simulink model "ps1"  (R2020b)
settings: Solver=VariableStepAuto  StartTime=0.0  StopTime=10.0  RelTol=1e-3
undefined symbols (not defined in the file): b, K1, k12, M1, M2
settings Model: Creator=prana  LastModifiedBy=prana

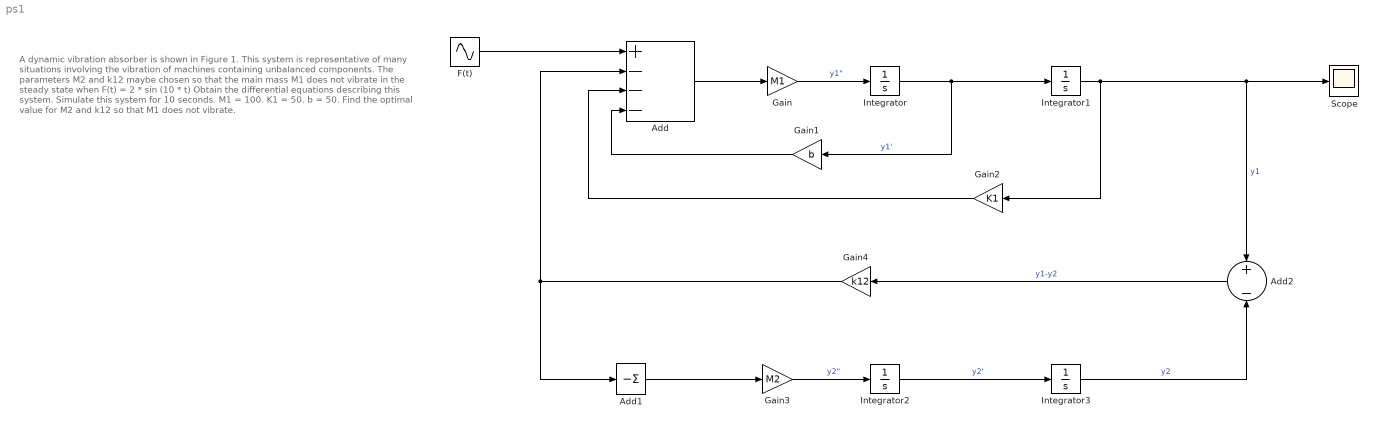
== system ps1 ==
  note: A dynamic vibration absorber is shown in Figure 1. This system is representative of many situations involving the vibration of machines containing unbalanced components. The parameters M2 and k12 maybe chosen so that the main mass M1 does not vibrate in the steady state when F(t) = 2 * sin (10 * t) Obtain the differential equations describing this system. Simulate this system for 10 seconds. M1 = 100. K1 = 50. b = 50. Find the optimal value for M2 and k12 so that M1 does not vibrate.
  Add : Sum  Inputs=+---
  Add1 : Sum  Inputs=-
  Add2 : Sum  Inputs=+-
  F(t) : Sin  Amplitude=2  Frequency=10  SampleTime=0
  Gain : Gain  Gain=M1
  Gain1 : Gain  Gain=b
  Gain2 : Gain  Gain=K1
  Gain3 : Gain  Gain=M2
  Gain4 : Gain  Gain=k12
  Integrator{,1..3} (4 alike) : Integrator
  Scope : Scope
  wires:
  Integrator/1 -> Gain1/1, Integrator1/1  "y1'"
  Gain/1 -> Integrator/1  "y1\""
  Add/1 -> Gain/1
  F(t)/1 -> Add/1
  Integrator1/1 -> Gain2/1, Scope/1, Add2/1  "y1"
  Gain1/1 -> Add/4
  Gain2/1 -> Add/3
  Integrator2/1 -> Integrator3/1  "y2'"
  Gain3/1 -> Integrator2/1  "y2\""
  Integrator3/1 -> Add2/2  "y2"
  Add2/1 -> Gain4/1  "y1-y2"
  Add1/1 -> Gain3/1
  Gain4/1 -> Add/2, Add1/1
